simulink model "expt_non_holonomic"  (R2021a)
settings: Solver=VariableStepAuto  StartTime=0.0  StopTime=30  RelTol=1e-3
libraries: simulink x1
settings Model: Creator=dhruv  LastModifiedBy=dhruv

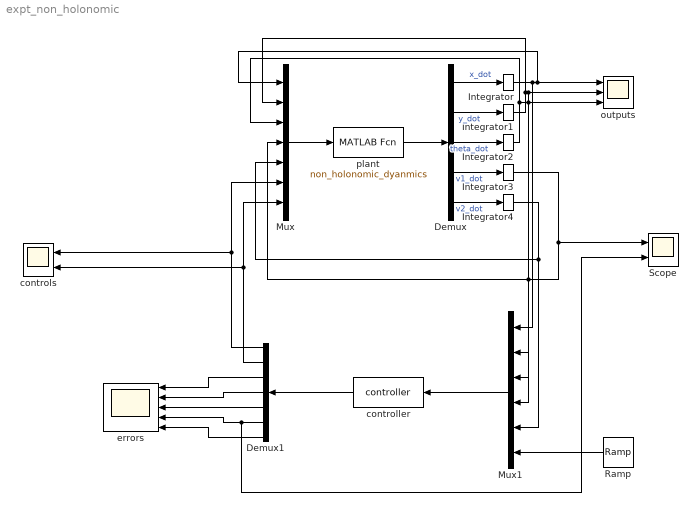
== system expt_non_holonomic ==
  Demux : Demux  Outputs=5
  Demux1 : Demux  Outputs=7
  Integrator : Integrator  InitialCondition=-1
  Integrator1 : Integrator  InitialCondition=2
  Integrator2 : Integrator  InitialCondition=pi/4
  Integrator3 : Integrator
  Integrator4 : Integrator
  Mux : Mux  Inputs=7
  Mux1 : Mux  Inputs=6
  Ramp : simulink/Sources/Ramp  slope=5  start=0  InitialOutput=0
  Scope : Scope  NumInputPorts=2
  controller : MATLABFcn  MATLABFcn=controller  OutputDimensions=7
  controls : Scope  NumInputPorts=2
  errors : Scope  NumInputPorts=5
  outputs : Scope  NumInputPorts=3
  plant : MATLABFcn  MATLABFcn=non_holonomic_dyanmics  OutputDimensions=5
  wires:
  Mux/1 -> plant/1
  plant/1 -> Demux/1
  Demux/1 -> Integrator/1  "x_dot"
  Demux/2 -> Integrator1/1  "y_dot"
  Demux/3 -> Integrator2/1  "theta_dot"
  Demux/4 -> Integrator3/1  "v1_dot"
  Demux/5 -> Integrator4/1  "v2_dot"
  Integrator/1 -> outputs/1, Mux/1, Mux1/1
  Integrator1/1 -> Mux1/2, outputs/2, Mux/2
  Integrator2/1 -> Mux1/3, outputs/3, Mux/3
  Integrator3/1 -> Mux1/4, Mux/4, Scope/1
  Integrator4/1 -> Mux1/5, Mux/5
  Mux1/1 -> controller/1
  Ramp/1 -> Mux1/6
  controller/1 -> Demux1/1
  Demux1/1 -> controls/1, Mux/6
  Demux1/2 -> Mux/7, controls/2
  Demux1/3 -> errors/1
  Demux1/4 -> errors/2
  Demux1/5 -> errors/3
  Demux1/6 -> Scope/2, errors/4
  Demux1/7 -> errors/5
